simulink model "Full_Ride_Model"  (R2025b)
settings: Solver=VariableStepAuto  StartTime=0.0  StopTime=10  MaxStep=0.001  RelTol=1e-3
values from neighbouring files (symbols this model uses):
  a = L - b    (= 0.8525)    [Susp_and_wheel_load_modelling.m]
  b = wf * L    (= 0.6975)    [Susp_and_wheel_load_modelling.m]
libraries: SignalEditorBlockLib x1
settings Model: Creator=CAM  LastModifiedBy=CAM
settings DebuggingCC: UnderSpecifiedDimensionMsg=warning

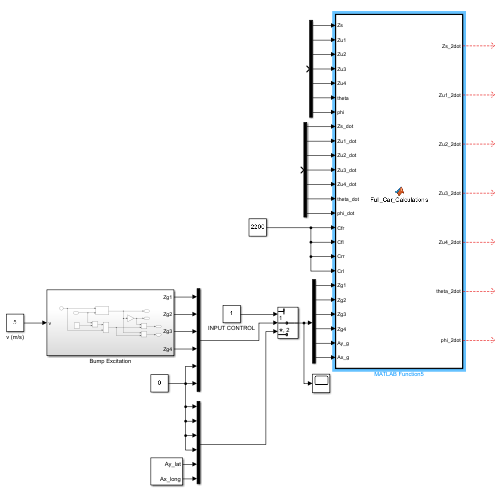
[thumbnail: Simulink's stored preview of the top-level diagram]
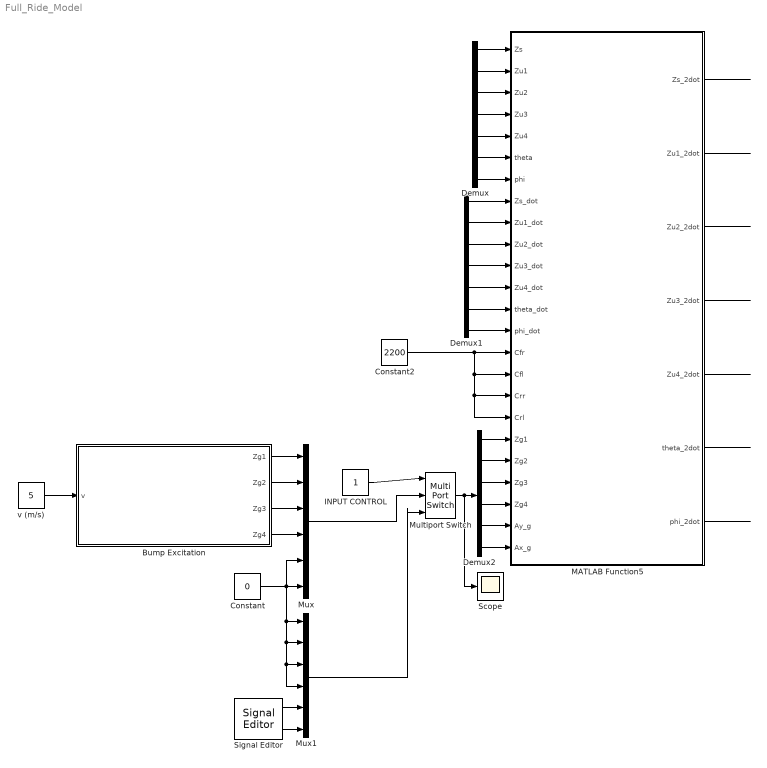
== system Full_Ride_Model ==
  Bump Excitation : Subsystem
  Constant : Constant  Value=0
  Constant2 : Constant  Value=2200
  Demux : Demux  Outputs=7
  Demux1 : Demux  Outputs=7
  Demux2 : Demux  Outputs=6
  INPUT CONTROL : Constant
  MATLAB Function5 : MATLAB Function  TreatAsAtomicUnit=on
  Multiport Switch : MultiPortSwitch  Inputs=2  SaturateOnIntegerOverflow=off  InputSameDT=off
  Mux : Mux  Inputs=6
  Mux1 : Mux  Inputs=6
  Scope : Scope
      settings: ActiveDisplayYMinimum=-0.0058356614738691208  ActiveDisplayYMaximum=0.025747888492856825
  Signal Editor : SignalEditorBlockLib/Signal Editor  FileName=road_excitations.mat  ActiveScenario=Scenario1  ActiveSignal=Ay_lat  IsBus=off  OutputBusObjectStr=Bus: BusObject  SampleTime=-1  ZeroCross=off  OutputAfterFinalValue=Setting to zero  Unit=inherit  PreserveSignalName=on  ApplySigPropsToAllScenarios=on  ApplySigPropsToAllSignals=on  SignalPropertySource=Dialog parameters
  v (m/s) : Constant  Value=5
  wires:
  MATLAB Function5/4(Zu3_2dot) -> ?
  MATLAB Function5/6(theta_2dot) -> ?
  Constant2/1 -> MATLAB Function5/18(Crl), MATLAB Function5/17(Crr), MATLAB Function5/16(Cfl), MATLAB Function5/15(Cfr)
  Demux/1 -> MATLAB Function5/1(Zs)
  Demux/2 -> MATLAB Function5/2(Zu1)
  Demux/3 -> MATLAB Function5/3(Zu2)
  Demux/4 -> MATLAB Function5/4(Zu3)
  Demux/5 -> MATLAB Function5/5(Zu4)
  Demux/6 -> MATLAB Function5/6(theta)
  Demux/7 -> MATLAB Function5/7(phi)
  Demux1/1 -> MATLAB Function5/8(Zs_dot)
  Demux1/2 -> MATLAB Function5/9(Zu1_dot)
  Demux1/3 -> MATLAB Function5/10(Zu2_dot)
  Demux1/4 -> MATLAB Function5/11(Zu3_dot)
  Demux1/5 -> MATLAB Function5/12(Zu4_dot)
  Demux1/6 -> MATLAB Function5/13(theta_dot)
  Demux1/7 -> MATLAB Function5/14(phi_dot)
  MATLAB Function5/3(Zu2_2dot) -> ?
  MATLAB Function5/2(Zu1_2dot) -> ?
  MATLAB Function5/5(Zu4_2dot) -> ?
  MATLAB Function5/7(phi_2dot) -> ?
  MATLAB Function5/1(Zs_2dot) -> ?
  Mux1/1 -> Multiport Switch/3
  Mux/1 -> Multiport Switch/2
  Multiport Switch/1 -> Scope/1, Demux2/1
  Demux2/1 -> MATLAB Function5/19(Zg1)
  Demux2/2 -> MATLAB Function5/20(Zg2)
  Demux2/3 -> MATLAB Function5/21(Zg3)
  Demux2/4 -> MATLAB Function5/22(Zg4)
  Demux2/5 -> MATLAB Function5/23(Ay_g)
  Demux2/6 -> MATLAB Function5/24(Ax_g)
  v (m/s)/1 -> Bump Excitation/1(v)
  Bump Excitation/1(Zg1) -> Mux/1
  Bump Excitation/2(Zg2) -> Mux/2
  Bump Excitation/3(Zg3) -> Mux/3
  Bump Excitation/4(Zg4) -> Mux/4
  Constant/1 -> Mux1/4, Mux1/3, Mux1/2, Mux1/1, Mux/5, Mux/6
  INPUT CONTROL/1 -> Multiport Switch/1
  Signal Editor/1 -> Mux1/5
  Signal Editor/2 -> Mux1/6

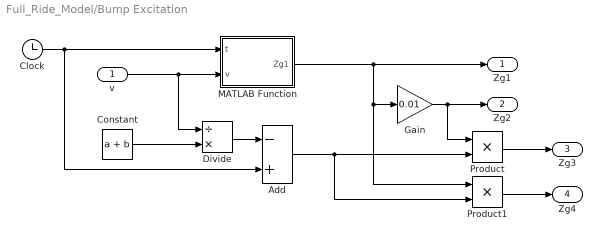
== system Full_Ride_Model/Bump Excitation ==
  v : Inport
  Add : Sum  Inputs=-+
  Clock : Clock
  Constant : Constant  Value=a + b
  Divide : Product  Inputs=/*
  Gain : Gain  Gain=0.01
  MATLAB Function : MATLAB Function  TreatAsAtomicUnit=on
  Product : Product
  Product1 : Product
  Zg1 : Outport
  Zg2 : Outport  Port=2
  Zg3 : Outport  Port=3
  Zg4 : Outport  Port=4
  wires:
  Gain/1 -> Zg2/1, Product/1
  Add/1 -> Product1/2, Product/2
  MATLAB Function/1(Zg1) -> Zg1/1, Product1/1, Gain/1
  Product/1 -> Zg3/1
  Clock/1 -> Add/2, MATLAB Function/1(t)
  Product1/1 -> Zg4/1
  v/1 -> Divide/1, MATLAB Function/2(v)
  Constant/1 -> Divide/2
  Divide/1 -> Add/1

== matlab function Full_Ride_Model/Bump Excitation/MATLAB Function ==
  data: t input; Zg1 output; v input
function Zg1 = fcn(t, v)
    H = 0.1;       % Height of bump (meters)
    L = 0.50;       % Length of bump (meters)
    T_start = 2.0;  % Start time (seconds)

    % Calculate distance traveled into the bump
    d = v * (t - T_start);

    % Check if the car is currently over the bump length
    if (d > 0) && (d < L)
        % Generate the hump (0 to Pi is the positive half of a sine wave)
        Zg1 = H * sin(pi * d / L);
    else
        % Flat road everywhere else
        Zg1 = 0;
    end
end

== matlab function Full_Ride_Model/MATLAB Function5 ==
  data: Zs input; Zu1 input; Zu2 input; Zu3 input; Zu4 input; theta input; phi input; Zs_2dot output; Zs_dot input; Zu1_2dot output; Zu1_dot input; Zu2_dot input; Zu3_dot input; Zu4_dot input; theta_dot input; phi_dot input; Cfr input; Cfl input; Crr input; Crl input; Zg1 input; Zg2 input; Zg3 input; Zg4 input; Zu2_2dot output; Zu3_2dot output; Zu4_2dot output; theta_2dot output; phi_2dot output; Ay_g input; Ax_g input
function [Zs_2dot, Zu1_2dot, Zu2_2dot, Zu3_2dot, Zu4_2dot, theta_2dot, phi_2dot] = Full_Car_Calculations(Zs, Zu1, Zu2, Zu3, Zu4, theta, phi, Zs_dot, Zu1_dot, Zu2_dot, Zu3_dot, Zu4_dot, theta_dot, phi_dot, Cfr, Cfl, Crr, Crl, Zg1, Zg2, Zg3, Zg4, Ay_g, Ax_g)
 
    ksf = 43.78 * 1000; 
    ksr = 43.78 * 1000; 
    kt  = 120 * 1000;   
    
    Mu = 50;       
    Ms = 250;      
    h = 0.325;%CG Height (m)
    
    % Mass Per Corner
    m_corner_f = (Mu * 0.45) / 2; 
    m_corner_r = (Mu * 0.55) / 2; 
    
    L = 1.55;      
    wf = 0.45;     
    b = wf * L;    
    a = L - b;     
    
    tf = 1.250;    
    tr = 1.200;    
    w_f = tf / 2;  
    w_r = tr / 2;  
    
    avg_width = (tf + tr) / 2;
    Ixx = 1/12 * Ms * (avg_width^2);  
    Iyy = 1/12 * Ms * (L^2);          
    
    % --- MOMENTS FROM G-FORCE ---
    % Convert G's to m/s^2
    Ay = Ay_g * 9.81;
    Ax = Ax_g * 9.81;

    % Roll Moment (Force * Moment Arm)
    % Lat Force acts at Ground, Inertia at CG. Arm = h.
    % Positive Ay (Turning Left) -> Centrifugal Force pushes Right -> Roll Positive
    M_roll_inertial = Ms * Ay * h;

    % Pitch Moment
    % Positive Ax (Acceleration) -> Inertia pushes Back -> Nose Up (Theta -)
    % Negative Ax (Braking) -> Inertia pushes Forward -> Nose Down (Theta +)
    % Note: Check your Theta sign convention. If Theta+ is Nose Down:
    M_pitch_inertial = -Ms * Ax * h; 

    % --- FORCES (Same as before) ---
    Fks1 = ksf * (Zu1 + a*theta + w_f*phi - Zs);
    Fc1  = Cfr * (Zu1_dot + a*theta_dot + w_f*phi_dot - Zs_dot);
    
    Fks2 = ksf * (Zu2 + a*theta - w_f*phi - Zs);
    Fc2  = Cfl * (Zu2_dot + a*theta_dot - w_f*phi_dot - Zs_dot);
    
    Fks3 = ksr * (Zu3 - b*theta + w_r*phi - Zs); 
    Fc3  = Crr * (Zu3_dot - b*theta_dot + w_r*phi_dot - Zs_dot);
    
    Fks4 = ksr * (Zu4 - b*theta - w_r*phi - Zs);
    Fc4  = Crl * (Zu4_dot - b*theta_dot - w_r*phi_dot - Zs_dot);

    % --- ACCELERATIONS ---
    Zu1_2dot = ( kt*(Zg1 - Zu1) - Fks1 - Fc1 ) / m_corner_f;
    Zu2_2dot = ( kt*(Zg2 - Zu2) - Fks2 - Fc2 ) / m_corner_f;
    Zu3_2dot = ( kt*(Zg3 - Zu3) - Fks3 - Fc3 ) / m_corner_r;
    Zu4_2dot = ( kt*(Zg4 - Zu4) - Fks4 - Fc4 ) / m_corner_r;
    
    Zs_2dot = ((Fks1 + Fc1 + Fks2 + Fc2 + Fks3 + Fc3 + Fks4 + Fc4) / Ms); 
    
    % Add Inertial Roll Moment to the suspension moments
    phi_2dot = ((Fks2 + Fc2)*w_f + (Fks4 + Fc4)*w_r - (Fks3 + Fc3)*w_r - (Fks1 + Fc1)*w_f + M_roll_inertial) / Ixx;
    
    % Add Inertial Pitch Moment to the suspension moments
    theta_2dot = ((Fks4 + Fc4)*b + (Fks3 + Fc3)*b - (Fks2 + Fc2)*a - (Fks1 + Fc1)*a + M_pitch_inertial) / Iyy;
end
